simulink model "quad_1_ref_NN_ports_cex_R2016a"  (R2016a)
settings: Solver=FixedStepAuto  SolverMode=SingleTasking  StartTime=0.0  StopTime=20  FixedStep=0.01  RelTol=1e-3
libraries: neural x348, simulink x2
(part 3 of 13)

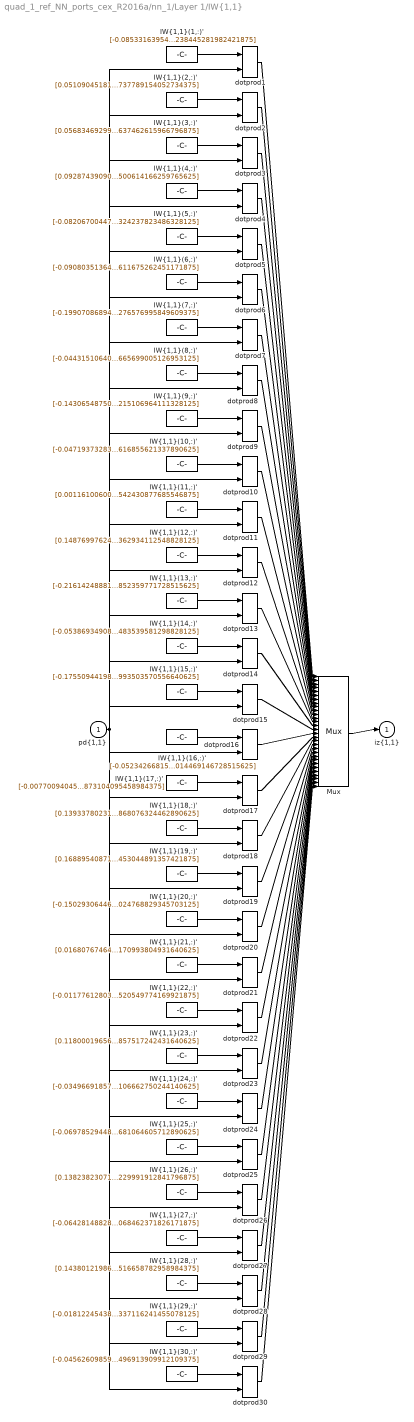
== system quad_1_ref_NN_ports_cex_R2016a/nn_1/Layer 1/IW{1,1} ==
  "pd{1,1}" : Inport  PortDimensions=12
      mask Display: e = 0.06;c1 = [120 230 180]/255;c2 = ([120 230 180]+0)/(256+128);c3 = ([120 230 180]+128)/(256+128);patch([0 1 1 0],[0 0 1 1],c1);patch([0 1 1 1-e 1-e 0+e],[0 0 1 1-e 0+e 0+e],c2);patch([0 0 1 1-e 0+e 0+e],[0 1 1 1-e 1-e 0+e],c3);plot([0 1 1 0 0],[0 0 1 1 0]);
  "IW{1,1}(1,:)'" : Constant  Value=[-0.08533163954011911689345737386247492395341396331787109375;0.023701383699620541534169859687608550302684307098388671875;-0.00984524590033421416468417675105229136534035205841064453125;0.08838272475303483866060361151539837010204792022705078125;-0.00624274279006867445496187229991846834309399127960205078125;0.0215454831971510878119158149957002024166285991668701171875;-0.046864654791841153791409624318475835025310516357421875;-0.021537524585770677354457092178563470952212810516357421875;-0.0294734818935463611933034400180986267514526844024658203125;0.004322611923815261776582463681961598922498524188995361328125;-0.010335355978819009414859664275354589335620403289794921875;0.0108123401776163800824814842371779377572238445281982421875]
      mask Display: e = 0.06;c1 = [120 150 230]/255;c2 = ([120 150 230]+0)/383;c3 = ([120 150 230]+128)/383;patch([0 1 1 0],[0 0 1 1],c1);patch([0 1 1 1-e 1-e 0+e],[0 0 1 1-e 0+e 0+e],c2);patch([0 0 1 1-e 0+e 0+e],[0 1 1 1-e 1-e 0+e],c3);plot([0 1 1 0 0],[0 0 1 1 0]);disp('Weights');
  "IW{1,1}(10,:)'" : Constant  Value=[-0.04719373283639781424536607801201171241700649261474609375;0.010986797568800034385905206590905436314642429351806640625;0.0099968896067782302139459460477155516855418682098388671875;0.043526614154225783115403913825502968393266201019287109375;-0.0214445197523684093210416534702744684182107448577880859375;0.015547049474153980253010587375683826394379138946533203125;0.01013989018363679883716343965716077946126461029052734375;0.00099486849642584605779571660377769148908555507659912109375;-0.033379999032854108798051839812615071423351764678955078125;0.0234671400648791272924853501535835675895214080810546875;0.00912580354643799385172542315558530390262603759765625;0.00791420646163809582418480204069055616855621337890625]
      mask Display: e = 0.06;c1 = [120 150 230]/255;c2 = ([120 150 230]+0)/383;c3 = ([120 150 230]+128)/383;patch([0 1 1 0],[0 0 1 1],c1);patch([0 1 1 1-e 1-e 0+e],[0 0 1 1-e 0+e 0+e],c2);patch([0 0 1 1-e 0+e 0+e],[0 1 1 1-e 1-e 0+e],c3);plot([0 1 1 0 0],[0 0 1 1 0]);disp('Weights');
  "IW{1,1}(11,:)'" : Constant  Value=[0.001161006005616034564287275543392752297222614288330078125;0.0282752717692778161862054986386283417232334613800048828125;0.0082830969855650533884006136986499768681824207305908203125;-0.0799271556537590466273712763722869567573070526123046875;0.03514083377957356868481753053856664337217807769775390625;-0.0350050314058179823373251338125555776059627532958984375;0.00551296932723115314101125505885647726245224475860595703125;0.0205416185189068699334935530487200594507157802581787109375;0.0109178870885326684270211217153700999915599822998046875;0.0270865660417085700462092034968009102158248424530029296875;0.00604959229913186631588661867908740532584488391876220703125;0.016624224988253326340537086025506141595542430877685546875]
      mask Display: e = 0.06;c1 = [120 150 230]/255;c2 = ([120 150 230]+0)/383;c3 = ([120 150 230]+128)/383;patch([0 1 1 0],[0 0 1 1],c1);patch([0 1 1 1-e 1-e 0+e],[0 0 1 1-e 0+e 0+e],c2);patch([0 0 1 1-e 0+e 0+e],[0 1 1 1-e 1-e 0+e],c3);plot([0 1 1 0 0],[0 0 1 1 0]);disp('Weights');
  "IW{1,1}(12,:)'" : Constant  Value=[0.14876997624185384072603710592375136911869049072265625;-0.034084589957586015895873998715615016408264636993408203125;-0.01172043168386959453852735890677649877034127712249755859375;-0.2176666807682514359623127120357821695506572723388671875;-0.03274459495796989971783119699466624297201633453369140625;0.0417850220856566256788511282138642854988574981689453125;0.119623043338685508540919499864685349166393280029296875;-0.002633586945418931769824499866672340431250631809234619140625;-0.000164254421362816128981965135835707769729197025299072265625;-0.026556739080857115486988817565361387096345424652099609375;-0.03013978069456739461440264449265669099986553192138671875;0.01227107587700693343280011760043635149486362934112548828125]
      mask Display: e = 0.06;c1 = [120 150 230]/255;c2 = ([120 150 230]+0)/383;c3 = ([120 150 230]+128)/383;patch([0 1 1 0],[0 0 1 1],c1);patch([0 1 1 1-e 1-e 0+e],[0 0 1 1-e 0+e 0+e],c2);patch([0 0 1 1-e 0+e 0+e],[0 1 1 1-e 1-e 0+e],c3);plot([0 1 1 0 0],[0 0 1 1 0]);disp('Weights');
  "IW{1,1}(13,:)'" : Constant  Value=[-0.216142488810365851481520849119988270103931427001953125;-0.034586804365752711609705016826410428620874881744384765625;-0.0514941842448963793543725842027924954891204833984375;0.2451148519358883060004217213645461015403270721435546875;-0.0301120377669227730355050454136289772577583789825439453125;-0.007175654035724382713568036962215046514756977558135986328125;-0.1977303928165770885438945470014004968106746673583984375;0.027127115427833199678975262258973089046776294708251953125;0.034656943517482476091462473277715616859495639801025390625;-0.038595691725607027267042070661773323081433773040771484375;0.009086982071260817084290550837977207265794277191162109375;-0.0190588981703795935784828685655156732536852359771728515625]
      mask Display: e = 0.06;c1 = [120 150 230]/255;c2 = ([120 150 230]+0)/383;c3 = ([120 150 230]+128)/383;patch([0 1 1 0],[0 0 1 1],c1);patch([0 1 1 1-e 1-e 0+e],[0 0 1 1-e 0+e 0+e],c2);patch([0 0 1 1-e 0+e 0+e],[0 1 1 1-e 1-e 0+e],c3);plot([0 1 1 0 0],[0 0 1 1 0]);disp('Weights');
  "IW{1,1}(14,:)'" : Constant  Value=[-0.053869349089182193279778942951452336274087429046630859375;0.003237690873636361703347130713837032089941203594207763671875;0.0163403794449467586191726553579428582452237606048583984375;0.025163165053367082812929567126047913916409015655517578125;0.0035123919087605391664563825315781286917626857757568359375;-0.00317408702623861622982293084760385681875050067901611328125;0.00402828104663707255161941844789907918311655521392822265625;0.0157539866788296671618052613439431297592818737030029296875;-0.0122787115338949155696202097942659747786819934844970703125;0.02707247382610743213771087312125018797814846038818359375;0.0099068320438581679299172577657373039983212947845458984375;-0.015680949750953750154724986032306333072483539581298828125]
      mask Display: e = 0.06;c1 = [120 150 230]/255;c2 = ([120 150 230]+0)/383;c3 = ([120 150 230]+128)/383;patch([0 1 1 0],[0 0 1 1],c1);patch([0 1 1 1-e 1-e 0+e],[0 0 1 1-e 0+e 0+e],c2);patch([0 0 1 1-e 0+e 0+e],[0 1 1 1-e 1-e 0+e],c3);plot([0 1 1 0 0],[0 0 1 1 0]);disp('Weights');
  "IW{1,1}(15,:)'" : Constant  Value=[-0.1755094419822800233532689162530004978179931640625;-0.0318393515554545036838618443653103895485401153564453125;-0.0351752783743397301474686855726758949458599090576171875;0.19963109579440863061705613290541805326938629150390625;0.0014567333978588968557144056603647186420857906341552734375;0.01162177621180309795845264630997917265631258487701416015625;-0.05078117076653558548127165295227314345538616180419921875;-0.0011086586167863205810990567812268636771477758884429931640625;-0.00821564631056164763889260171936257393099367618560791015625;-0.020409472758647510814977721338436822406947612762451171875;-0.038221513076739821457294965512119233608245849609375;-0.036013450461401787239257288320004590786993503570556640625]
      mask Display: e = 0.06;c1 = [120 150 230]/255;c2 = ([120 150 230]+0)/383;c3 = ([120 150 230]+128)/383;patch([0 1 1 0],[0 0 1 1],c1);patch([0 1 1 1-e 1-e 0+e],[0 0 1 1-e 0+e 0+e],c2);patch([0 0 1 1-e 0+e 0+e],[0 1 1 1-e 1-e 0+e],c3);plot([0 1 1 0 0],[0 0 1 1 0]);disp('Weights');
  "IW{1,1}(16,:)'" : Constant  Value=[-0.05234266815478318124466028393726446665823459625244140625;0.0163295409455364026740653571323491632938385009765625;0.0184565486566411925128949889085561153478920459747314453125;0.025899139837868102864693042874932871200144290924072265625;-0.02601451939107861377475927611158112995326519012451171875;0.011476195623872954831856674218215630389750003814697265625;-0.00358947245972765331678555611460978980176150798797607421875;-0.01539670123886757550912829373146450961939990520477294921875;-0.0344596196305909929780142419986077584326267242431640625;0.00470461014677240295378535250847562565468251705169677734375;0.00069603480178562367707006952599613214260898530483245849609375;0.019492938385435122639055549598197103478014469146728515625]
      mask Display: e = 0.06;c1 = [120 150 230]/255;c2 = ([120 150 230]+0)/383;c3 = ([120 150 230]+128)/383;patch([0 1 1 0],[0 0 1 1],c1);patch([0 1 1 1-e 1-e 0+e],[0 0 1 1-e 0+e 0+e],c2);patch([0 0 1 1-e 0+e 0+e],[0 1 1 1-e 1-e 0+e],c3);plot([0 1 1 0 0],[0 0 1 1 0]);disp('Weights');
  "IW{1,1}(17,:)'" : Constant  Value=[-0.007700940458927864329385926112081506289541721343994140625;-0.0142473278132610285673376182558058644644916057586669921875;0.014336036410234724580714527064628782682120800018310546875;0.0475688149083226818891745324435760267078876495361328125;-0.014008638151867432164454640997064416296780109405517578125;0.013050130965458262011225087917409837245941162109375;0.0054159603812769831210349735783893265761435031890869140625;-0.0134663012546911188549447757623056531883776187896728515625;-0.011599545947326726780257644122684723697602748870849609375;0.012427405935565190298053295236968551762402057647705078125;0.0107474512119018310307705377226739074103534221649169921875;-0.02251448850870418905145697863190434873104095458984375]
      mask Display: e = 0.06;c1 = [120 150 230]/255;c2 = ([120 150 230]+0)/383;c3 = ([120 150 230]+128)/383;patch([0 1 1 0],[0 0 1 1],c1);patch([0 1 1 1-e 1-e 0+e],[0 0 1 1-e 0+e 0+e],c2);patch([0 0 1 1-e 0+e 0+e],[0 1 1 1-e 1-e 0+e],c3);plot([0 1 1 0 0],[0 0 1 1 0]);disp('Weights');
  "IW{1,1}(18,:)'" : Constant  Value=[0.139337802311172709313069617564906366169452667236328125;0.01522622847992911691850093092170936870388686656951904296875;-0.002272157029607591895159490746891606249846518039703369140625;-0.265583206080534151016792066002381034195423126220703125;-0.013642761818601085999080879673783783800899982452392578125;0.0021848175936124251961256703680192003957927227020263671875;0.1754777672786185516162760222869110293686389923095703125;0.015002173038253706349731686486848047934472560882568359375;-0.0107229780998079095299946317254580208100378513336181640625;0.004251767945528228676010940034757368266582489013671875;-0.02216784377437831798918210779447690583765506744384765625;0.0030644068720353835610925585797303938306868076324462890625]
      mask Display: e = 0.06;c1 = [120 150 230]/255;c2 = ([120 150 230]+0)/383;c3 = ([120 150 230]+128)/383;patch([0 1 1 0],[0 0 1 1],c1);patch([0 1 1 1-e 1-e 0+e],[0 0 1 1-e 0+e 0+e],c2);patch([0 0 1 1-e 0+e 0+e],[0 1 1 1-e 1-e 0+e],c3);plot([0 1 1 0 0],[0 0 1 1 0]);disp('Weights');
  "IW{1,1}(19,:)'" : Constant  Value=[0.168895408715680372946366105679771862924098968505859375;0.00796289105770174067411293350460255169309675693511962890625;-0.023381887980152303574410410647033131681382656097412109375;-0.1396617157085457139320538999527343548834323883056640625;-0.0166680235096560540319909904383166576735675334930419921875;0.008446022533223296324678130986285395920276641845703125;0.059529269021017135188333924133985419757664203643798828125;-0.014092144936405558153236228235982707701623439788818359375;-0.027933581023289529021713661904868786223232746124267578125;-0.01675003665652145812270390479170600883662700653076171875;-0.027816197436945890031356753979707718826830387115478515625;0.00839144223413626315355440254961649770848453044891357421875]
      mask Display: e = 0.06;c1 = [120 150 230]/255;c2 = ([120 150 230]+0)/383;c3 = ([120 150 230]+128)/383;patch([0 1 1 0],[0 0 1 1],c1);patch([0 1 1 1-e 1-e 0+e],[0 0 1 1-e 0+e 0+e],c2);patch([0 0 1 1-e 0+e 0+e],[0 1 1 1-e 1-e 0+e],c3);plot([0 1 1 0 0],[0 0 1 1 0]);disp('Weights');
  "IW{1,1}(2,:)'" : Constant  Value=[0.051090451818023123464751478195466916076838970184326171875;0.001327907848030623720603227155834247241728007793426513671875;0.001844152968076073241532331081771189928986132144927978515625;-0.031831381917390190461336629823563271202147006988525390625;-0.0079942003085606942736074387312328326515853404998779296875;-0.0235101337779398920913020987200070521794259548187255859375;0.00199225618291611235310956118382819113321602344512939453125;0.0255197443792113017047018530547575210221111774444580078125;0.0263347497737178616594722058152910904027521610260009765625;-0.0240783408578300432700824984522114391438663005828857421875;-0.00658503837704377086026408250063468585722148418426513671875;0.0145734689246425040687338281486518098972737789154052734375]
      mask Display: e = 0.06;c1 = [120 150 230]/255;c2 = ([120 150 230]+0)/383;c3 = ([120 150 230]+128)/383;patch([0 1 1 0],[0 0 1 1],c1);patch([0 1 1 1-e 1-e 0+e],[0 0 1 1-e 0+e 0+e],c2);patch([0 0 1 1-e 0+e 0+e],[0 1 1 1-e 1-e 0+e],c3);plot([0 1 1 0 0],[0 0 1 1 0]);disp('Weights');
  "IW{1,1}(20,:)'" : Constant  Value=[-0.15029306446958312637462995553505606949329376220703125;-0.0052998707162357737432412108091739355586469173431396484375;-0.028765229709817784209402447004322311840951442718505859375;0.185818755084005304833993932334124110639095306396484375;-0.018986003761860888172652295224906993098556995391845703125;-0.00751328152694412214340768940701309475116431713104248046875;-0.037383823504194502174158287743921391665935516357421875;0.01559091004442587045930590505804502754472196102142333984375;-0.00330872425771615817635673550967112532816827297210693359375;0.0017391487430674749947723256582321482710540294647216796875;-0.004699281656393654305059470743799465708434581756591796875;-0.0062033523970312816342431716520877671428024768829345703125]
      mask Display: e = 0.06;c1 = [120 150 230]/255;c2 = ([120 150 230]+0)/383;c3 = ([120 150 230]+128)/383;patch([0 1 1 0],[0 0 1 1],c1);patch([0 1 1 1-e 1-e 0+e],[0 0 1 1-e 0+e 0+e],c2);patch([0 0 1 1-e 0+e 0+e],[0 1 1 1-e 1-e 0+e],c3);plot([0 1 1 0 0],[0 0 1 1 0]);disp('Weights');
  "IW{1,1}(21,:)'" : Constant  Value=[0.016807674645452484740726362133500515483319759368896484375;-0.01886425913792307007543769259427790530025959014892578125;-0.007994033265164866841612223424817784689366817474365234375;0.0061379424463088340380156893161256448365747928619384765625;-0.0170021270007992865436197149620056734420359134674072265625;0.01187593788226888082137921998082674690522253513336181640625;0.004313867250208221204577085927667212672531604766845703125;0.0198375276912271247820029884678660891950130462646484375;0.019758925309838019923613927630867692641913890838623046875;0.0099178306100423142821487232367871911264955997467041015625;-0.0161297819820095979237439820508370758034288883209228515625;0.0004860381828146491584898003512904551826068200170993804931640625]
      mask Display: e = 0.06;c1 = [120 150 230]/255;c2 = ([120 150 230]+0)/383;c3 = ([120 150 230]+128)/383;patch([0 1 1 0],[0 0 1 1],c1);patch([0 1 1 1-e 1-e 0+e],[0 0 1 1-e 0+e 0+e],c2);patch([0 0 1 1-e 0+e 0+e],[0 1 1 1-e 1-e 0+e],c3);plot([0 1 1 0 0],[0 0 1 1 0]);disp('Weights');
  "IW{1,1}(22,:)'" : Constant  Value=[-0.0117761280335450697898114214012821321375668048858642578125;-0.007381325083734278404146156304932446801103651523590087890625;0.01039595251946430660983100580097016063518822193145751953125;0.00837663755954763146471808710202822112478315830230712890625;0.0235007717290987468150564865254636970348656177520751953125;-0.0119102049258410606913383134042305755428969860076904296875;-0.00413221782339760930480299094824658823199570178985595703125;0.022591689367830687651395038528789882548153400421142578125;0.005517940269701540438596065740739504690282046794891357421875;-0.018299449669380761507309074431759654544293880462646484375;0.010881354047579137878098975988905294798314571380615234375;-0.0193488810930286074529771411789624835364520549774169921875]
      mask Display: e = 0.06;c1 = [120 150 230]/255;c2 = ([120 150 230]+0)/383;c3 = ([120 150 230]+128)/383;patch([0 1 1 0],[0 0 1 1],c1);patch([0 1 1 1-e 1-e 0+e],[0 0 1 1-e 0+e 0+e],c2);patch([0 0 1 1-e 0+e 0+e],[0 1 1 1-e 1-e 0+e],c3);plot([0 1 1 0 0],[0 0 1 1 0]);disp('Weights');
  "IW{1,1}(23,:)'" : Constant  Value=[0.1180001965623702908647629783445154316723346710205078125;-0.01375682072700455844949107842012381297536194324493408203125;-0.0354938780843749857041302675497718155384063720703125;-0.1813898567265349315302813693051575683057308197021484375;-0.003959884089565455199399846009100656374357640743255615234375;-0.0007001210349296231594262707176312687806785106658935546875;0.07568545327198535066504092583272722549736499786376953125;-0.016186387356645660917653373189750709570944309234619140625;0.0160660583402277568065841251154779456555843353271484375;-0.0279952650117144714869699129167202045209705829620361328125;-0.004537226985211174901113651003470295108854770660400390625;-0.0202533201691001731037378164046458550728857517242431640625]
      mask Display: e = 0.06;c1 = [120 150 230]/255;c2 = ([120 150 230]+0)/383;c3 = ([120 150 230]+128)/383;patch([0 1 1 0],[0 0 1 1],c1);patch([0 1 1 1-e 1-e 0+e],[0 0 1 1-e 0+e 0+e],c2);patch([0 0 1 1-e 0+e 0+e],[0 1 1 1-e 1-e 0+e],c3);plot([0 1 1 0 0],[0 0 1 1 0]);disp('Weights');
  "IW{1,1}(24,:)'" : Constant  Value=[-0.03496691857278010073795115886241546832025051116943359375;0.007748338021483981707948629491511383093893527984619140625;-0.0026083095597784337373037377716400442295707762241363525390625;0.0169618925426850593318750526350413565523922443389892578125;0.0129595070011701805900994344256105250678956508636474609375;0.0106744444151387028740796125703127472661435604095458984375;0.0113921693664603036755256226797428098507225513458251953125;-0.0086266177395414415929320028908477979712188243865966796875;0.020386534787887773678694003365308162756264209747314453125;0.007799054091837322177926949962056824006140232086181640625;-0.010097139118999308438073825300307362340390682220458984375;0.016755972256266883635422715315144159831106662750244140625]
      mask Display: e = 0.06;c1 = [120 150 230]/255;c2 = ([120 150 230]+0)/383;c3 = ([120 150 230]+128)/383;patch([0 1 1 0],[0 0 1 1],c1);patch([0 1 1 1-e 1-e 0+e],[0 0 1 1-e 0+e 0+e],c2);patch([0 0 1 1-e 0+e 0+e],[0 1 1 1-e 1-e 0+e],c3);plot([0 1 1 0 0],[0 0 1 1 0]);disp('Weights');
  "IW{1,1}(25,:)'" : Constant  Value=[-0.0697852944862396018521621954278089106082916259765625;0.0241347190606308568960880478471153764985501766204833984375;0.030239508647953043662948147130009601823985576629638671875;0.1384098074059808280988903561592451296746730804443359375;0.0094173570316700982996138691305532120168209075927734375;0.0111211637250735219384356611271869041956961154937744140625;-0.051420816851884217080215222495098714716732501983642578125;0.00142578007845343447679287152141114347614347934722900390625;0.0123955914408080715427562523700544261373579502105712890625;0.0297157792056183499285193505556890158914029598236083984375;0.00967658513736770718727253637325702584348618984222412109375;-0.01518476032294514832532428272315883077681064605712890625]
      mask Display: e = 0.06;c1 = [120 150 230]/255;c2 = ([120 150 230]+0)/383;c3 = ([120 150 230]+128)/383;patch([0 1 1 0],[0 0 1 1],c1);patch([0 1 1 1-e 1-e 0+e],[0 0 1 1-e 0+e 0+e],c2);patch([0 0 1 1-e 0+e 0+e],[0 1 1 1-e 1-e 0+e],c3);plot([0 1 1 0 0],[0 0 1 1 0]);disp('Weights');
  "IW{1,1}(26,:)'" : Constant  Value=[0.1382382307132225263135438808603794313967227935791015625;-0.01149466037825518961723592070711674750782549381256103515625;0.0253576523672179275636917594738406478427350521087646484375;-0.1267515379637365047216235325322486460208892822265625;-0.01021131967257968807538670574786010547541081905364990234375;-0.01026520638173537836035364989584195427596569061279296875;0.06437717127772658864959254287896328605711460113525390625;0.004907467909692362663387488197486163699068129062652587890625;0.011255985110878281851842785954431747086346149444580078125;0.0132604501975320289430815279274611384607851505279541015625;-0.00141489613489247773557566656421613515703938901424407958984375;-0.0052099784673837017112685288111606496386229991912841796875]
      mask Display: e = 0.06;c1 = [120 150 230]/255;c2 = ([120 150 230]+0)/383;c3 = ([120 150 230]+128)/383;patch([0 1 1 0],[0 0 1 1],c1);patch([0 1 1 1-e 1-e 0+e],[0 0 1 1-e 0+e 0+e],c2);patch([0 0 1 1-e 0+e 0+e],[0 1 1 1-e 1-e 0+e],c3);plot([0 1 1 0 0],[0 0 1 1 0]);disp('Weights');
  "IW{1,1}(27,:)'" : Constant  Value=[-0.06428148828106201861931623398049850948154926300048828125;0.0059147217569273762005632733007587376050651073455810546875;0.01750994443044305570733598642618744634091854095458984375;0.047929126939194301171287548868349404074251651763916015625;-0.0033064674184476706107760346498025683104060590267181396484375;0.0126082770843921020131883636850034235976636409759521484375;0.01236916216500257015287189688024227507412433624267578125;0.0115842782371548651265680263122703763656318187713623046875;-0.00151471954015441716279166683989387820474803447723388671875;0.027595876742433932127251949850688106380403041839599609375;0.003886387407313164794875337548774041351862251758575439453125;0.01157854824893300542398844044100769679062068462371826171875]
      mask Display: e = 0.06;c1 = [120 150 230]/255;c2 = ([120 150 230]+0)/383;c3 = ([120 150 230]+128)/383;patch([0 1 1 0],[0 0 1 1],c1);patch([0 1 1 1-e 1-e 0+e],[0 0 1 1-e 0+e 0+e],c2);patch([0 0 1 1-e 0+e 0+e],[0 1 1 1-e 1-e 0+e],c3);plot([0 1 1 0 0],[0 0 1 1 0]);disp('Weights');
  "IW{1,1}(28,:)'" : Constant  Value=[0.1438012198622841408823802566985250450670719146728515625;-0.018719716038484490727711317958892323076725006103515625;0.00513472849813346836345129275969156879000365734100341796875;-0.1808535758183016095568262926462921313941478729248046875;-0.0296601682541367296652712326476830639876425266265869140625;0.00691847219015410963560697155116940848529338836669921875;0.0574548780329277863909709367362665943801403045654296875;0.002886354409094356310294671175142866559326648712158203125;0.01033067302177755053538277252300758846104145050048828125;0.016584129398255716136834081453343969769775867462158203125;-0.022137833269114580436731642976155853830277919769287109375;-0.000620296331590392512056464369152308790944516658782958984375]
      mask Display: e = 0.06;c1 = [120 150 230]/255;c2 = ([120 150 230]+0)/383;c3 = ([120 150 230]+128)/383;patch([0 1 1 0],[0 0 1 1],c1);patch([0 1 1 1-e 1-e 0+e],[0 0 1 1-e 0+e 0+e],c2);patch([0 0 1 1-e 0+e 0+e],[0 1 1 1-e 1-e 0+e],c3);plot([0 1 1 0 0],[0 0 1 1 0]);disp('Weights');
  "IW{1,1}(29,:)'" : Constant  Value=[-0.018122454387302942835358265938339172862470149993896484375;-0.017222250065498823090592850348912179470062255859375;-0.0144314176181656421416032998195078107528388500213623046875;0.03294853384948488728145576942551997490227222442626953125;-0.0158701554005997967633501133377649239264428615570068359375;0.020135494385374812231770391690588439814746379852294921875;-0.016183316384210742755467293818583129905164241790771484375;-0.01283954643310499139918778865876447525806725025177001953125;-0.017642140324184964195186609003940247930586338043212890625;0.004527395050893574975081623534833852318115532398223876953125;-0.0018374316771737468113878666287064334028400480747222900390625;-0.0182825547733219302692919683295258437283337116241455078125]
      mask Display: e = 0.06;c1 = [120 150 230]/255;c2 = ([120 150 230]+0)/383;c3 = ([120 150 230]+128)/383;patch([0 1 1 0],[0 0 1 1],c1);patch([0 1 1 1-e 1-e 0+e],[0 0 1 1-e 0+e 0+e],c2);patch([0 0 1 1-e 0+e 0+e],[0 1 1 1-e 1-e 0+e],c3);plot([0 1 1 0 0],[0 0 1 1 0]);disp('Weights');
  "IW{1,1}(3,:)'" : Constant  Value=[0.05683469299552383613427508635140839032828807830810546875;-0.003565981349764761609844043732664431445300579071044921875;-0.018185489295623913363897372619248926639556884765625;-0.1780806771733315085892712659187964163720607757568359375;0.0187960506062180600361788407326457672752439975738525390625;-0.028625094132411856018283202729435288347303867340087890625;0.07407559484627114498866973235635668970644474029541015625;-0.0029850992708978681122733433994653751142323017120361328125;0.0200508845041174367518355126094320439733564853668212890625;-0.0106044024886904585114333343653925112448632717132568359375;-0.0019468629914965000782256510092338430695235729217529296875;0.0072692701345010816982306067757235723547637462615966796875]
      mask Display: e = 0.06;c1 = [120 150 230]/255;c2 = ([120 150 230]+0)/383;c3 = ([120 150 230]+128)/383;patch([0 1 1 0],[0 0 1 1],c1);patch([0 1 1 1-e 1-e 0+e],[0 0 1 1-e 0+e 0+e],c2);patch([0 0 1 1-e 0+e 0+e],[0 1 1 1-e 1-e 0+e],c3);plot([0 1 1 0 0],[0 0 1 1 0]);disp('Weights');
  "IW{1,1}(30,:)'" : Constant  Value=[-0.045626098593807014325296478318705339916050434112548828125;-0.0141314039407378945478743759167628013528883457183837890625;-0.0006495663615152728713464380660980168613605201244354248046875;0.03063644807732164576652422738334280438721179962158203125;-0.0096495936185285492714402977298959740437567234039306640625;0.016031264085592002166524849826600984670221805572509765625;-0.0081837514413762059428680828432334237731993198394775390625;0.01942351432130295929567864732234738767147064208984375;0.0073101569482917246045605708104631048627197742462158203125;-0.0116708612966481724282363785505367559380829334259033203125;-0.01053572333116568372768373507142314338125288486480712890625;0.0191387028324687367974998863928703940473496913909912109375]
      mask Display: e = 0.06;c1 = [120 150 230]/255;c2 = ([120 150 230]+0)/383;c3 = ([120 150 230]+128)/383;patch([0 1 1 0],[0 0 1 1],c1);patch([0 1 1 1-e 1-e 0+e],[0 0 1 1-e 0+e 0+e],c2);patch([0 0 1 1-e 0+e 0+e],[0 1 1 1-e 1-e 0+e],c3);plot([0 1 1 0 0],[0 0 1 1 0]);disp('Weights');
  "IW{1,1}(4,:)'" : Constant  Value=[0.09287439090355363580098213560631847940385341644287109375;0.00921974170501765714902386861240302096121013164520263671875;0.0050356940348545153884884939543553628027439117431640625;-0.11225030076966525938164664921714575029909610748291015625;0.004367058229483906754697652985441891360096633434295654296875;-0.01221041751807180712752209927884905482642352581024169921875;0.05291791666845944985819727435227832756936550140380859375;0.00517278028422177814371618609357028617523610591888427734375;0.01550058320354012926511888537106642615981400012969970703125;0.00900711115333137531113738560861747828312218189239501953125;0.0174367615481985094305628081201575696468353271484375;0.009581004430800045545968401938807801343500614166259765625]
      mask Display: e = 0.06;c1 = [120 150 230]/255;c2 = ([120 150 230]+0)/383;c3 = ([120 150 230]+128)/383;patch([0 1 1 0],[0 0 1 1],c1);patch([0 1 1 1-e 1-e 0+e],[0 0 1 1-e 0+e 0+e],c2);patch([0 0 1 1-e 0+e 0+e],[0 1 1 1-e 1-e 0+e],c3);plot([0 1 1 0 0],[0 0 1 1 0]);disp('Weights');
  "IW{1,1}(5,:)'" : Constant  Value=[-0.08206700447948621357507903439909568987786769866943359375;0.0159598316208878938937676394971276749856770038604736328125;0.0260527096603565093413390485466152313165366649627685546875;0.06760178954245298077463388608521199785172939300537109375;0.00948444513378582897134005946782053797505795955657958984375;0.018262351887242130044075594241803628392517566680908203125;-0.023292971586573112119378237139244447462260723114013671875;-0.0232729844218795868526772352424814016558229923248291015625;-0.0154500295853803037982032719810376875102519989013671875;0.0152295757405039901277721270389520213939249515533447265625;-0.018733878123929507963918439372719149105250835418701171875;0.005139268109960443316197586938187669147737324237823486328125]
      mask Display: e = 0.06;c1 = [120 150 230]/255;c2 = ([120 150 230]+0)/383;c3 = ([120 150 230]+128)/383;patch([0 1 1 0],[0 0 1 1],c1);patch([0 1 1 1-e 1-e 0+e],[0 0 1 1-e 0+e 0+e],c2);patch([0 0 1 1-e 0+e 0+e],[0 1 1 1-e 1-e 0+e],c3);plot([0 1 1 0 0],[0 0 1 1 0]);disp('Weights');
  "IW{1,1}(6,:)'" : Constant  Value=[-0.09080351364880796805056917264664662070572376251220703125;0.0253694379929296671971616916607672465033829212188720703125;0.007852166291116215168788272649180726148188114166259765625;0.0710749511246341614256749608102836646139621734619140625;0.0142695719516449277819436503023098339326679706573486328125;-0.00481443946506703024379447697356226854026317596435546875;-0.047118953830480890532239612866760580800473690032958984375;-0.036981233657886920795920815407953341491520404815673828125;-0.0420038949462573640847296019273926503956317901611328125;0.01352807829769145202269964300967330927960574626922607421875;-0.01086400930026619644774843465029334765858948230743408203125;-0.00711880762028205098246314008747503976337611675262451171875]
      mask Display: e = 0.06;c1 = [120 150 230]/255;c2 = ([120 150 230]+0)/383;c3 = ([120 150 230]+128)/383;patch([0 1 1 0],[0 0 1 1],c1);patch([0 1 1 1-e 1-e 0+e],[0 0 1 1-e 0+e 0+e],c2);patch([0 0 1 1-e 0+e 0+e],[0 1 1 1-e 1-e 0+e],c3);plot([0 1 1 0 0],[0 0 1 1 0]);disp('Weights');
  "IW{1,1}(7,:)'" : Constant  Value=[-0.1990708689499143257961577546666376292705535888671875;-0.002149132181086997606112021230728714726865291595458984375;-0.0176719389875768344289053146667356486432254314422607421875;0.1612323918629600949525837449982645921409130096435546875;-0.00135096369008205242912001864397097961045801639556884765625;0.00963436255806263998346938848271747701801359653472900390625;-0.1259379831659615811556562903206213377416133880615234375;0.0247657028951250961223973234837103518657386302947998046875;0.00967374046263661142852630092647814308293163776397705078125;0.01130288450982687431523032728364341892302036285400390625;0.0038937517866595959536990534388678497634828090667724609375;-0.01446578023452270433946154071236378513276576995849609375]
      mask Display: e = 0.06;c1 = [120 150 230]/255;c2 = ([120 150 230]+0)/383;c3 = ([120 150 230]+128)/383;patch([0 1 1 0],[0 0 1 1],c1);patch([0 1 1 1-e 1-e 0+e],[0 0 1 1-e 0+e 0+e],c2);patch([0 0 1 1-e 0+e 0+e],[0 1 1 1-e 1-e 0+e],c3);plot([0 1 1 0 0],[0 0 1 1 0]);disp('Weights');
  "IW{1,1}(8,:)'" : Constant  Value=[-0.04431510640925122312960837689388426952064037322998046875;0.006452880059851100018331049312791947158984839916229248046875;-0.0021979860508054664680610557070394861511886119842529296875;0.09368262680619056370634467612035223282873630523681640625;0.0021070523193057431876606955256647779606282711029052734375;0.0173501247713280411233416344884972204454243183135986328125;-0.020527887335963800052862637812722823582589626312255859375;-0.00596978907006493093867494081905533676035702228546142578125;0.00465803052872669660910975863998828572221100330352783203125;0.015792971159140682668731159310482325963675975799560546875;-0.0161436225807279794264292860361820203252136707305908203125;-0.0106922331328965121433061113975782063789665699005126953125]
      mask Display: e = 0.06;c1 = [120 150 230]/255;c2 = ([120 150 230]+0)/383;c3 = ([120 150 230]+128)/383;patch([0 1 1 0],[0 0 1 1],c1);patch([0 1 1 1-e 1-e 0+e],[0 0 1 1-e 0+e 0+e],c2);patch([0 0 1 1-e 0+e 0+e],[0 1 1 1-e 1-e 0+e],c3);plot([0 1 1 0 0],[0 0 1 1 0]);disp('Weights');
  "IW{1,1}(9,:)'" : Constant  Value=[-0.1430654875005125947762252280881511978805065155029296875;0.022072060034107200687802929905956261791288852691650390625;-0.003911074725607386302905776886973399086855351924896240234375;0.18769677232603687588863294877228327095508575439453125;0.00498574486860386099917885616150670102797448635101318359375;-0.002213016074695960296037089420906340819783508777618408203125;-0.0902890257440757959539467947251978330314159393310546875;0.01344929035273954680274055561994828167371451854705810546875;-0.01280990901107668424041552412973032915033400058746337890625;0.0212321649887824148716930494629195891320705413818359375;0.029870647420559968965303454524473636411130428314208984375;0.0210110208466124555315435173952209879644215106964111328125]
      mask Display: e = 0.06;c1 = [120 150 230]/255;c2 = ([120 150 230]+0)/383;c3 = ([120 150 230]+128)/383;patch([0 1 1 0],[0 0 1 1],c1);patch([0 1 1 1-e 1-e 0+e],[0 0 1 1-e 0+e 0+e],c2);patch([0 0 1 1-e 0+e 0+e],[0 1 1 1-e 1-e 0+e],c3);plot([0 1 1 0 0],[0 0 1 1 0]);disp('Weights');
  Mux : Mux  Inputs=30
      mask Display: e = 0.06;c1 = [120 150 230]/255;c2 = ([120 150 230]+0)/383;c3 = ([120 150 230]+128)/383;patch([0 1 1 0],[0 0 1 1],c1);patch([0 1 1 1-e 1-e 0+e],[0 0 1 1-e 0+e 0+e],c2);patch([0 0 1 1-e 0+e 0+e],[0 1 1 1-e 1-e 0+e],c3);plot([0 1 1 0 0],[0 0 1 1 0]);disp('Mux');
  dotprod{1..30} (30 alike) : neural/Weight Functions/dotprod
  "iz{1,1}" : Outport
      mask Display: e = 0.06;c1 = [120 230 180]/255;c2 = ([120 230 180]+0)/(256+128);c3 = ([120 230 180]+128)/(256+128);patch([0 1 1 0],[0 0 1 1],c1);patch([0 1 1 1-e 1-e 0+e],[0 0 1 1-e 0+e 0+e],c2);patch([0 0 1 1-e 0+e 0+e],[0 1 1 1-e 1-e 0+e],c3);plot([0 1 1 0 0],[0 0 1 1 0]);
  wires:
  "IW{1,1}(1,:)'"/1 -> dotprod1/1
  "pd{1,1}"/1 -> dotprod1/2, dotprod2/2, dotprod3/2, dotprod4/2, dotprod5/2, dotprod6/2, dotprod7/2, dotprod8/2, dotprod9/2, dotprod10/2, dotprod11/2, dotprod12/2, dotprod13/2, dotprod14/2, dotprod15/2, dotprod16/2, dotprod17/2, dotprod18/2, dotprod19/2, dotprod20/2, dotprod21/2, dotprod22/2, dotprod23/2, dotprod24/2, dotprod25/2, dotprod26/2, dotprod27/2, dotprod28/2, dotprod29/2, dotprod30/2
  dotprod1/1 -> Mux/1
  "IW{1,1}(2,:)'"/1 -> dotprod2/1
  dotprod2/1 -> Mux/2
  "IW{1,1}(3,:)'"/1 -> dotprod3/1
  dotprod3/1 -> Mux/3
  "IW{1,1}(4,:)'"/1 -> dotprod4/1
  dotprod4/1 -> Mux/4
  "IW{1,1}(5,:)'"/1 -> dotprod5/1
  dotprod5/1 -> Mux/5
  "IW{1,1}(6,:)'"/1 -> dotprod6/1
  dotprod6/1 -> Mux/6
  "IW{1,1}(7,:)'"/1 -> dotprod7/1
  dotprod7/1 -> Mux/7
  "IW{1,1}(8,:)'"/1 -> dotprod8/1
  dotprod8/1 -> Mux/8
  "IW{1,1}(9,:)'"/1 -> dotprod9/1
  dotprod9/1 -> Mux/9
  "IW{1,1}(10,:)'"/1 -> dotprod10/1
  dotprod10/1 -> Mux/10
  "IW{1,1}(11,:)'"/1 -> dotprod11/1
  dotprod11/1 -> Mux/11
  "IW{1,1}(12,:)'"/1 -> dotprod12/1
  dotprod12/1 -> Mux/12
  "IW{1,1}(13,:)'"/1 -> dotprod13/1
  dotprod13/1 -> Mux/13
  "IW{1,1}(14,:)'"/1 -> dotprod14/1
  dotprod14/1 -> Mux/14
  "IW{1,1}(15,:)'"/1 -> dotprod15/1
  dotprod15/1 -> Mux/15
  "IW{1,1}(16,:)'"/1 -> dotprod16/1
  dotprod16/1 -> Mux/16
  "IW{1,1}(17,:)'"/1 -> dotprod17/1
  dotprod17/1 -> Mux/17
  "IW{1,1}(18,:)'"/1 -> dotprod18/1
  dotprod18/1 -> Mux/18
  "IW{1,1}(19,:)'"/1 -> dotprod19/1
  dotprod19/1 -> Mux/19
  "IW{1,1}(20,:)'"/1 -> dotprod20/1
  dotprod20/1 -> Mux/20
  "IW{1,1}(21,:)'"/1 -> dotprod21/1
  dotprod21/1 -> Mux/21
  "IW{1,1}(22,:)'"/1 -> dotprod22/1
  dotprod22/1 -> Mux/22
  "IW{1,1}(23,:)'"/1 -> dotprod23/1
  dotprod23/1 -> Mux/23
  "IW{1,1}(24,:)'"/1 -> dotprod24/1
  dotprod24/1 -> Mux/24
  "IW{1,1}(25,:)'"/1 -> dotprod25/1
  dotprod25/1 -> Mux/25
  "IW{1,1}(26,:)'"/1 -> dotprod26/1
  dotprod26/1 -> Mux/26
  "IW{1,1}(27,:)'"/1 -> dotprod27/1
  dotprod27/1 -> Mux/27
  "IW{1,1}(28,:)'"/1 -> dotprod28/1
  dotprod28/1 -> Mux/28
  "IW{1,1}(29,:)'"/1 -> dotprod29/1
  dotprod29/1 -> Mux/29
  "IW{1,1}(30,:)'"/1 -> dotprod30/1
  dotprod30/1 -> Mux/30
  Mux/1 -> "iz{1,1}"/1

== system quad_1_ref_NN_ports_cex_R2016a/nn_1/Layer 2/Delays 1 ==
  "p{2}" : Inport  PortDimensions=30
      mask Display: e = 0.06;c1 = [120 230 180]/255;c2 = ([120 230 180]+0)/(256+128);c3 = ([120 230 180]+128)/(256+128);patch([0 1 1 0],[0 0 1 1],c1);patch([0 1 1 1-e 1-e 0+e],[0 0 1 1-e 0+e 0+e],c2);patch([0 0 1 1-e 0+e 0+e],[0 1 1 1-e 1-e 0+e],c3);plot([0 1 1 0 0],[0 0 1 1 0]);
  mux : Mux  Inputs=1
      mask Display: e = 0.06;c1 = [120 150 230]/255;c2 = ([120 150 230]+0)/383;c3 = ([120 150 230]+128)/383;patch([0 1 1 0],[0 0 1 1],c1);patch([0 1 1 1-e 1-e 0+e],[0 0 1 1-e 0+e 0+e],c2);patch([0 0 1 1-e 0+e 0+e],[0 1 1 1-e 1-e 0+e],c3);plot([0 1 1 0 0],[0 0 1 1 0]);disp('Mux')
  "pd{2,1}" : Outport
      mask Display: e = 0.06;c1 = [120 230 180]/255;c2 = ([120 230 180]+0)/(256+128);c3 = ([120 230 180]+128)/(256+128);patch([0 1 1 0],[0 0 1 1],c1);patch([0 1 1 1-e 1-e 0+e],[0 0 1 1-e 0+e 0+e],c2);patch([0 0 1 1-e 0+e 0+e],[0 1 1 1-e 1-e 0+e],c3);plot([0 1 1 0 0],[0 0 1 1 0]);
  wires:
  "p{2}"/1 -> mux/1
  mux/1 -> "pd{2,1}"/1
